simulink model "Lab4_Ex1"  (R2021a)
settings: Solver=VariableStepAuto  StartTime=0.0  StopTime=10.0  RelTol=1e-3
libraries: simulink x1
settings Model: Creator=student  LastModifiedBy=student

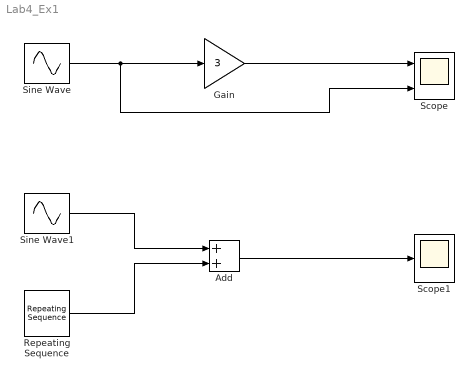
== system Lab4_Ex1 ==
  Add : Sum
  Gain : Gain  Gain=3
  Repeating Sequence : simulink/Sources/Repeating Sequence  rep_seq_t=[0 2]  rep_seq_y=[0 2]
  Scope : Scope  NumInputPorts=2
  Scope1 : Scope
  Sine Wave : Sin  SampleTime=0
  Sine Wave1 : Sin  SampleTime=0
  wires:
  Gain/1 -> Scope/1
  Sine Wave/1 -> Scope/2, Gain/1
  Add/1 -> Scope1/1
  Sine Wave1/1 -> Add/1
  Repeating Sequence/1 -> Add/2
